simulink model "sim_sil_top_TrapezoidalCommutation_s32k1xx"  (Simulink 9.0)
settings: Solver=FixedStepDiscrete  StartTime=0.0  StopTime=12  FixedStep=1  RelTol=1e-3  EnableMultiTasking=on
InitFcn:
  | mbd_s32k_consistency_checks(bdroot(gcs));
libraries: simulink x1
Description:
  | This model demonstrates the SIL concept. Using a HALL signal emulator the Trapezoidal Switching
  | algorithm is tested to ensure the proper PWM sequence is applied
  | 
  | Inputs:
  | - Rotation DIRECTION [CW(1) or CCW(-1)] can be set to 1(clockwise) or -1(counter clockwise).
  | - PWM duty cycle [PWM_Duty_Cycle] can be set to any value between 0-1.
  | 
  | Outputs:
  | Based on DIRECTION the comuttation sequence for each phase is updated.
  | - [Phase_A_HS] represents the computed PWM command for High Switch on Phase A
  | - [Phase_A_LS] represents the computed PWM command for Low Switch on Phase A
  | - [Phase_B_HS] represents the computed PWM command for High Switch on Phase B
  | - [Phase_B_LS] represents the computed PWM command for Low Switch on Phase B
  | - [Phase_C_HS] represents the computed PWM command for High Switch on Phase C
  | - [Phase_C_LS] represents the computed PWM command for Low Switch on Phase C
settings Model: Creator=NXP MBDT Team  LastModifiedBy=nxf35172
settings DataIOCC: ExternalInput=off  InitialState=off  LimitDataPoints=on  SaveOutput=off  SignalLogging=off  SaveTime=off
settings OptimizationCC: DefaultParameterBehavior=Inlined  EnhancedBackFolding=on  PassReuseOutputArgsAs=Individual arguments  LifeSpan=auto  OptimizeBlockOrder=speed  DifferentSizesBufferReuse=on
settings DebuggingCC: UnderspecifiedInitializationDetection=Simplified  MergeDetectMultiDrivingBlocksExec=error  SolverPrmCheckMsg=warning  InheritedTsInSrcMsg=none  SingleTaskRateTransMsg=error  ParameterTunabilityLossMsg=error  UnconnectedInputMsg=error  UnconnectedOutputMsg=error  UnconnectedLineMsg=error  AllowSymbolicDim=off  UnknownTsInhSupMsg=error
settings HardwareCC: ProdLargestAtomicInteger=Long  ProdLargestAtomicFloat=Double  ProdIntDivRoundTo=Zero  ProdEndianess=LittleEndian  ProdHWDeviceType=ARM Compatible->ARM Cortex
settings SFSimCC: MATLABDynamicMemAlloc=off
settings RTWCC: SystemTargetFile=mbd_s32k.tlc  MakeCommand=mbd_s32k_make_rtw COPY_MDLREF_INCLUDES=0  TemplateMakefile=mbd_s32k.tmf  Description=Model Based Design Toolbox S32K1xx Code Generation Target  GenerateReport=on  IncludeHyperlinkInReport=on  LaunchReport=on  PortableWordSizes=on  CreateSILPILBlock=PIL  GenerateTraceInfo=on  GenerateTraceReport=on  GenerateTraceReportSl=on  GenerateTraceReportSf=on  GenerateTraceReportEml=on
settings CodeAppCC: ForceParamTrailComments=on  IgnoreCustomStorageClasses=off  MaxIdLength=63  OperatorAnnotations=on  SimulinkDataObjDesc=on  SFDataObjDesc=on  InsertBlockDesc=on  StateflowObjectComments=off
settings STFCustomTargetCC: MultiwordLength=256  GenerateSampleERTMain=on  CombineOutputUpdateFcns=on  ERTCustomFileBanners=on  SupportContinuousTime=off  SupportNonInlinedSFcns=off  RemoveResetFunc=on  MATLABClassNameForMDSCustomization=Simulink.SoftwareTarget.ERTCustomization  GRTInterface=off  SystemTargetFile=mbd_s32k.tlc
settings ERTTargetCC: GenerateSampleERTMain=on  ParMdlRefBuildCompliant=off  CompOptLevelCompliant=off  ConcurrentExecutionCompliant=off  ModelStepFunctionPrototypeControlCompliant=off  CPPClassGenCompliant=off  UseToolchainInfoCompliant=off  InlinedParameterPlacement=NonHierarchical  ERTSrcFileBannerTemplate=mbd_ert_code_template.cgt  ERTHdrFileBannerTemplate=mbd_ert_code_template.cgt  ERTDataSrcFileTemplate=mbd_ert_code_template.cgt  ERTDataHdrFileTemplate=mbd_ert_code_template.cgt  ERTCustomFileTemplate=example_file_process.tlc

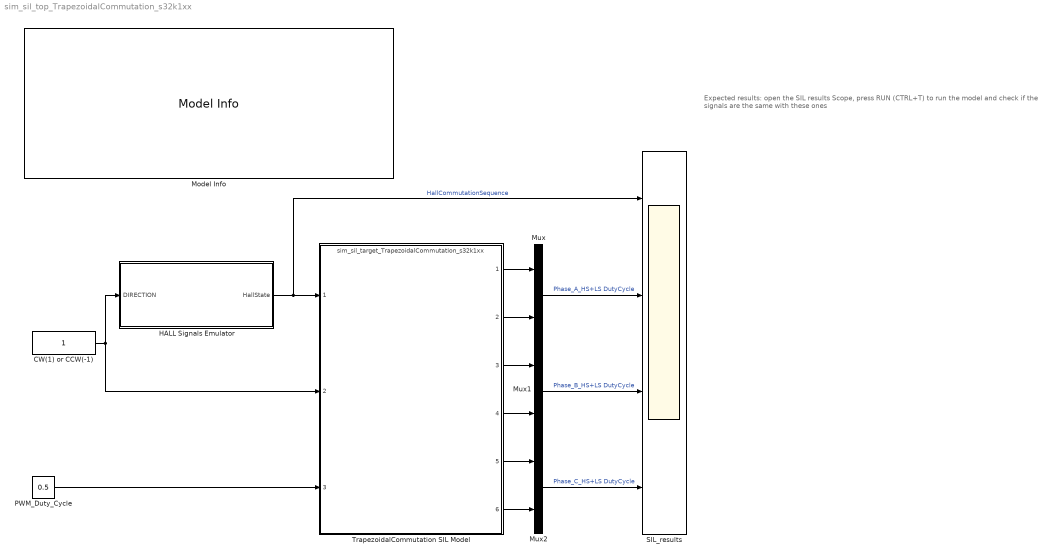
== system sim_sil_top_TrapezoidalCommutation_s32k1xx ==
  note: Expected results: open the SIL results Scope, press RUN (CTRL+T) to run the model and check
      | if the signals are the same with these ones
  CW(1) or CCW(-1) : Constant  OutMin=-1  OutMax=1  OutDataTypeStr=single
  HALL Signals Emulator : Subsystem
  Model Info : simulink/Model-Wide Utilities/Model Info  Frame=off  DisplayStringWithTags=|  HorizontalTextAlignment=Left  LeftAlignmentValue=0.02
      | Model Name: %<ModelName>
      | 
      | Description: %<Description>
  Mux : Mux  Inputs=2
  Mux1 : Mux  Inputs=2
  Mux2 : Mux  Inputs=2
  PWM_Duty_Cycle : Constant  Value=0.5  OutMin=0  OutMax=100  OutDataTypeStr=single
  SIL_results : Scope  NumInputPorts=4
  TrapezoidalCommutation SIL Model : ModelReference  ModelNameDialog=sim_sil_target_TrapezoidalCommutation_s32k1xx.mdl  SimulationMode=Software-in-the-loop (SIL)  ModelReferenceVersion=1.92
  wires:
  CW(1) or CCW(-1)/1 -> TrapezoidalCommutation SIL Model/2, HALL Signals Emulator/1(DIRECTION)
  PWM_Duty_Cycle/1 -> TrapezoidalCommutation SIL Model/3
  Mux/1 -> SIL_results/2  "Phase_A_HS+LS DutyCycle"
  TrapezoidalCommutation SIL Model/2 -> Mux/2
  TrapezoidalCommutation SIL Model/1 -> Mux/1
  TrapezoidalCommutation SIL Model/3 -> Mux1/1
  TrapezoidalCommutation SIL Model/4 -> Mux1/2
  Mux1/1 -> SIL_results/3  "Phase_B_HS+LS DutyCycle"
  TrapezoidalCommutation SIL Model/5 -> Mux2/1
  TrapezoidalCommutation SIL Model/6 -> Mux2/2
  Mux2/1 -> SIL_results/4  "Phase_C_HS+LS DutyCycle"
  HALL Signals Emulator/1(HallState) -> SIL_results/1, TrapezoidalCommutation SIL Model/1  "HallCommutationSequence"

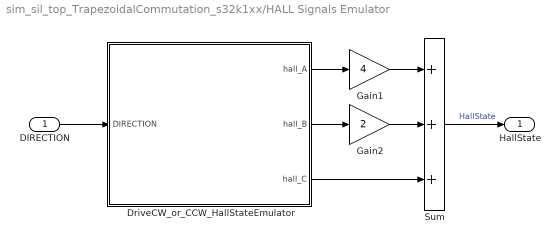
== system sim_sil_top_TrapezoidalCommutation_s32k1xx/HALL Signals Emulator ==
  DIRECTION : Inport
  DriveCW_or_CCW_HallStateEmulator : Stateflow chart  TreatAsAtomicUnit=on
  Gain1 : Gain  Gain=4  OutDataTypeStr=uint8  ParamDataTypeStr=Inherit: Same as input
  Gain2 : Gain  Gain=2  OutDataTypeStr=uint8  ParamDataTypeStr=Inherit: Same as input
  Sum : Sum  Inputs=+++  AccumDataTypeStr=uint8  OutDataTypeStr=uint8
  HallState : Outport
  wires:
  Sum/1 -> HallState/1  "HallState"
  Gain2/1 -> Sum/2
  DriveCW_or_CCW_HallStateEmulator/2(hall_B) -> Gain2/1
  Gain1/1 -> Sum/1
  DriveCW_or_CCW_HallStateEmulator/3(hall_C) -> Sum/3
  DriveCW_or_CCW_HallStateEmulator/1(hall_A) -> Gain1/1
  DIRECTION/1 -> DriveCW_or_CCW_HallStateEmulator/1(DIRECTION)

== stateflow chart HALL Signals Emulator/DriveCW_or_CCW_HallStateEmulator ==
  state STEP1
    entry:
    hall_A = uint8(1);
    hall_B = uint8(0);
    hall_C = uint8(0);
  state STEP2_CCW
    entry:
    hall_A = uint8(1);
    hall_B = uint8(0);
    hall_C = uint8(1);
  state STEP2_CW
    entry:
    hall_A = uint8(1);
    hall_B = uint8(1);
    hall_C = uint8(0);
  state STEP3_CCW
    entry:
    hall_A = uint8(0);
    hall_B = uint8(0);
    hall_C = uint8(1);
  state STEP3
    entry:
    hall_A = uint8(0);
    hall_B = uint8(1);
    hall_C = uint8(0);
  state STEP4_CCW
    entry:
    hall_A = uint8(0);
    hall_B = uint8(1);
    hall_C = uint8(1);
  state STEP4
    entry:
    hall_A = uint8(0);
    hall_B = uint8(1);
    hall_C = uint8(1);
  state STEP5_CCW
    entry:
    hall_A = uint8(0);
    hall_B = uint8(1);
    hall_C = uint8(0);
  state STEP5
    entry:
    hall_A = uint8(0);
    hall_B = uint8(0);
    hall_C = uint8(1);
  state STEP6_CCW
    entry:
    hall_A = uint8(1);
    hall_B = uint8(1);
    hall_C = uint8(0);
  state STEP6
    entry:
    hall_A = uint8(1);
    hall_B = uint8(0);
    hall_C = uint8(1);
  (default) -> STEP1
  STEP1 -> STEP2_CW [order 1] : [DIRECTION >=0]
  STEP1 -> STEP2_CCW [order 2] : [DIRECTION<0]
  STEP6_CCW -> STEP1
  STEP6 -> STEP1
  STEP2_CW -> STEP3
  STEP2_CCW -> STEP3_CCW
  STEP3_CCW -> STEP4_CCW
  STEP3 -> STEP4
  STEP4_CCW -> STEP5_CCW
  STEP4 -> STEP5
  STEP5_CCW -> STEP6_CCW
  STEP5 -> STEP6
  data: hall_A output uint8; hall_B output uint8; hall_C output uint8; DIRECTION input single
